simulink model "CryoDetHcd"  (R2016b)
settings: Solver=ode45  StartTime=0.0  StopTime=1e-3  RelTol=1e-3
PreLoadFcn:
  | setup_hcd
values from neighbouring files (symbols this model uses):
  A = sqrt(0.5*erfc(x))    [setup_hcd.m]
  Fadc = 307.2e6    (= 307200000)    [setupADCtoDACloopback.m]    (also in setupCryoFPGA_CMB.m; setup_hcd.m = 614000000)
undefined symbols (not defined in the file or in its folder): AXI4, B, C, D, etaRomData, freqRomData, freqRomData1, freqRomData2, freqRomData3, j, Lite
libraries: xbsIndex_r4 x897, CryoDetLibCMB x8, hdlsllib x8, dspsigops x2, simulink x1
(part 2 of 8)

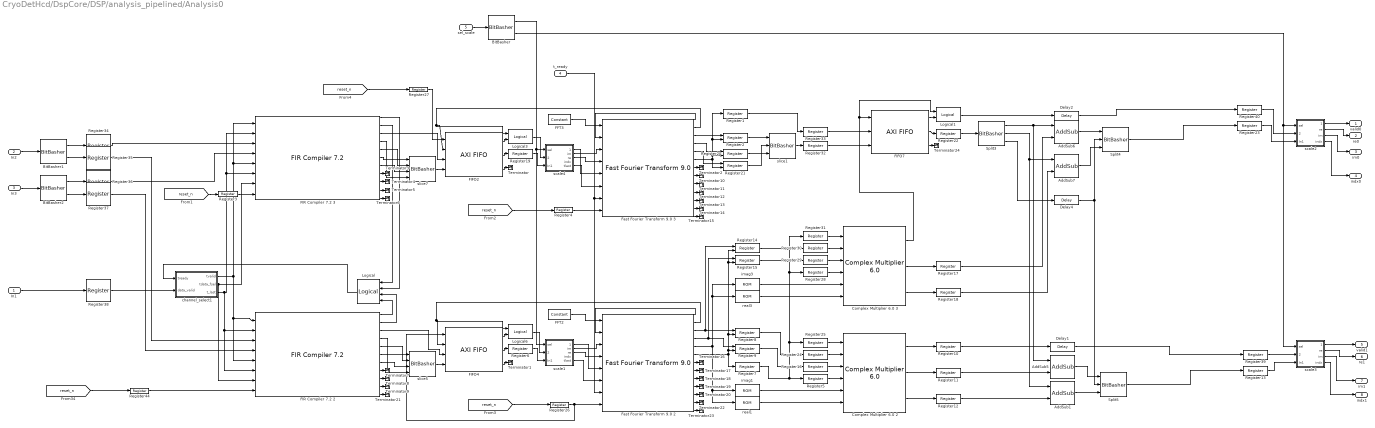
== system CryoDetHcd/DspCore/DSP/analysis_pipelined/Analysis0 ==
  In1 : Inport
  In2 : Inport  Port=2
  In3 : Inport  Port=3
  t_ready : Inport  Port=4
  sel_scale : Inport  Port=5
  AddSub{1,5..7} (4 alike) : xbsIndex_r4/AddSub  mode=Addition  use_carryin=off  use_carryout=off  en=off  latency=2  precision=Full  arith_type="Signed  (2's comp)"  n_bits=22  bin_pt=16  quantization=Truncate  overflow=Wrap  use_behavioral_HDL=on  hw_selection=Fabric  pipelined=off  dbl_ovrd=off  block_type=addsub
  BitBasher : xbsIndex_r4/BitBasher  bitexpr=|  display_expr=off  sr_1=sel0  arith_type1=Unsigned  bin_pt1=0  sr_2=sel1  arith_type2=Unsigned  bin_pt2=0  sr_3=3  arith_type3=Unsigned  bin_pt3=0  sr_4=4  arith_type4=Unsigned  bin_pt4=0  dbl_ovrd=off  block_type=bitbasher
      | sel0 = {in[0]}
      | sel1 = {in[1]}
  BitBasher1 : xbsIndex_r4/BitBasher  bitexpr=|  display_expr=off  sr_1=lo  arith_type1="Signed  (2's comp)"  bin_pt1=15  sr_2=hi  arith_type2="Signed  (2's comp)"  bin_pt2=15  sr_3=hi  arith_type3=Unsigned  bin_pt3=0  sr_4=4  arith_type4=Unsigned  bin_pt4=0  dbl_ovrd=off  block_type=bitbasher
      | lo = {in[15:0]}
      | hi = {in[31:16]}
  BitBasher2 : xbsIndex_r4/BitBasher  bitexpr=|  display_expr=off  sr_1=lo  arith_type1="Signed  (2's comp)"  bin_pt1=15  sr_2=hi  arith_type2="Signed  (2's comp)"  bin_pt2=15  sr_3=hi  arith_type3=Unsigned  bin_pt3=0  sr_4=4  arith_type4=Unsigned  bin_pt4=0  dbl_ovrd=off  block_type=bitbasher
      | lo = {in[15:0]}
      | hi = {in[31:16]}
  Complex Multiplier 6.0 2 : xbsIndex_r4/Complex Multiplier 6.0   hasatlast=off  hasatuser=off  atuserwidth=1  hasbtlast=off  hasbtuser=off  btuserwidth=1  multtype=Use_Mults  optimizegoal=Performance  flowcontrol=NonBlocking  outputwidth=24  roundmode=Truncate  hasctrltlast=off  hasctrltuser=off  ctrltuserwidth=1  outtlastbehv=Null  latencyconfig=Automatic  minimumlatency=34  aclken=off  aresetn=off  trim_axipin_name=on  simulation_type=hybrid_sim  simulation_model=sysgen:cmpy_v6_0  data_path_portlist={ 's_axis_a_tdata_real', 's_axis_a_tdata_imag', 's_axis_b_tdata_real', 's_axis_b_tdata_imag', 's_axis_ctrl_tdata_rounding_bit', 'm_axis_dout_tdata_real', 'm_axis_dout_tdata_imag' }  aportwidth=63  bportwidth=63  ip_name=Complex Multiplier  ip_version=6.0  dsptool_ready=true  ipcore_usecache=true  ipcore_useipmodelcache=true  ipcore_verbose=false  ipcore_latency_parameter='minimumlatency'  wrapper_available=true  port_translation_map={ 'aclken' => 'en', 'aresetn' => 'rst'}  block_type=cmpy_v6_0
  Complex Multiplier 6.0 3 : xbsIndex_r4/Complex Multiplier 6.0   hasatlast=off  hasatuser=off  atuserwidth=1  hasbtlast=off  hasbtuser=off  btuserwidth=1  multtype=Use_Mults  optimizegoal=Performance  flowcontrol=NonBlocking  outputwidth=24  roundmode=Truncate  hasctrltlast=off  hasctrltuser=off  ctrltuserwidth=1  outtlastbehv=Null  latencyconfig=Automatic  minimumlatency=34  aclken=off  aresetn=off  trim_axipin_name=on  simulation_type=hybrid_sim  simulation_model=sysgen:cmpy_v6_0  data_path_portlist={ 's_axis_a_tdata_real', 's_axis_a_tdata_imag', 's_axis_b_tdata_real', 's_axis_b_tdata_imag', 's_axis_ctrl_tdata_rounding_bit', 'm_axis_dout_tdata_real', 'm_axis_dout_tdata_imag' }  aportwidth=63  bportwidth=63  ip_name=Complex Multiplier  ip_version=6.0  dsptool_ready=true  ipcore_usecache=true  ipcore_useipmodelcache=true  ipcore_verbose=false  ipcore_latency_parameter='minimumlatency'  wrapper_available=true  port_translation_map={ 'aclken' => 'en', 'aresetn' => 'rst'}  block_type=cmpy_v6_0
  Delay1 : xbsIndex_r4/Delay  rst=off  infoeditControl=Selection of Reset will increase slice count due to use of real FFs and instead of SRLs  en=off  latency=2  reg_retiming=on  dbl_ovrd=off  block_type=delay
  Delay2 : xbsIndex_r4/Delay  rst=off  infoeditControl=Selection of Reset will increase slice count due to use of real FFs and instead of SRLs  en=off  latency=2  reg_retiming=on  dbl_ovrd=off  block_type=delay
  Delay4 : xbsIndex_r4/Delay  rst=off  infoeditControl=Selection of Reset will increase slice count due to use of real FFs and instead of SRLs  en=off  latency=2  reg_retiming=on  dbl_ovrd=off  block_type=delay
  FFT2 : xbsIndex_r4/Constant  const=1  gui_display_data_type=Fixed-point  arith_type=Unsigned  n_bits=1  bin_pt=0  preci_type=Single  exp_width=8  frac_width=24  explicit_period=off  period=1  equ=P=C  opselect=C  inp2=PCIN>>17  opr=+  inp1=P  carry=CIN  dbl_ovrd=off  block_type=constant
  FFT3 : xbsIndex_r4/Constant  const=1  gui_display_data_type=Fixed-point  arith_type=Unsigned  n_bits=1  bin_pt=0  preci_type=Single  exp_width=8  frac_width=24  explicit_period=off  period=1  equ=P=C  opselect=C  inp2=PCIN>>17  opr=+  inp1=P  carry=CIN  dbl_ovrd=off  block_type=constant
  FIFO2 : xbsIndex_r4/AXI FIFO  input_depth_axis=16  actual_fifo_depth_label=18  enable_tdata=on  enable_tdest=off  enable_tstrb=off  enable_tready=on  enable_tid=off  enable_tuser=off  enable_tkeep=off  enable_tlast=off  has_aresetn=on  enable_data_counts_axis=off  fifo_implementation_type_axis=Common Clock Distributed RAM  trim_axipin_name=on  programmable_full_type_axis=Full  full_threshold_assert_value_axis=0  programmable_empty_type_axis=Empty  empty_threshold_assert_value_axis=1022  underflow_flag_axi=0  underflow_sense_axi=Active High  overflow_flag_axi=0  overflow_sense_axi=Active High  block_type=axi_fifo
  FIFO4 : xbsIndex_r4/AXI FIFO  input_depth_axis=16  actual_fifo_depth_label=18  enable_tdata=on  enable_tdest=off  enable_tstrb=off  enable_tready=on  enable_tid=off  enable_tuser=off  enable_tkeep=off  enable_tlast=off  has_aresetn=on  enable_data_counts_axis=off  fifo_implementation_type_axis=Common Clock Distributed RAM  trim_axipin_name=on  programmable_full_type_axis=Full  full_threshold_assert_value_axis=0  programmable_empty_type_axis=Empty  empty_threshold_assert_value_axis=1022  underflow_flag_axi=0  underflow_sense_axi=Active High  overflow_flag_axi=0  overflow_sense_axi=Active High  block_type=axi_fifo
  FIFO7 : xbsIndex_r4/AXI FIFO  input_depth_axis=32  actual_fifo_depth_label=34  enable_tdata=on  enable_tdest=off  enable_tstrb=off  enable_tready=on  enable_tid=off  enable_tuser=off  enable_tkeep=off  enable_tlast=off  has_aresetn=off  enable_data_counts_axis=off  fifo_implementation_type_axis=Common Clock Distributed RAM  trim_axipin_name=on  programmable_full_type_axis=Full  full_threshold_assert_value_axis=0  programmable_empty_type_axis=Empty  empty_threshold_assert_value_axis=1022  underflow_flag_axi=0  underflow_sense_axi=Active High  overflow_flag_axi=0  overflow_sense_axi=Active High  block_type=axi_fifo
  FIR Compiler 7.2 2 : xbsIndex_r4/FIR Compiler 7.2   coefficientvector=analysis_coefficients2  coefficient_sets=8  coefficient_reload=off  filter_type=Single_Rate  rate_change_type=Integer  interpolation_rate=1  decimation_rate=1  zero_pack_factor=1  channel_sequence=Basic  number_channels=8  pattern_list='P4-0,P4-1,P4-2,P4-3,P4-4'  number_paths=2  ratespecification=Output_Sample_Period  sampleperiod=1.00000000  hardwareoversamplingrate=1  coefficient_sign=Signed  quantization=Quantize_Only  coefficient_width=25  bestprecision=on  coefficient_fractional_bits=28  coefficient_structure=Inferred  output_rounding_mode=Convergent_Rounding_to_Even  output_width=19  filter_architecture=Systolic_Multiply_Accumulate  optimization_goal=Area  optimization_list='None'  data_buffer_type=Automatic  coefficient_buffer_type=Automatic  input_buffer_type=Automatic  output_buffer_type=Automatic  preference_for_other_storage=Automatic  multi_column_support=Automatic  columnconfig='16'  inter_column_pipe_length=4  data_has_tlast=Vector_Framing  m_data_has_tready=off  s_data_has_fifo=off  s_data_has_tuser=Not_Required  m_data_has_tuser=Chan_ID_Field  s_config_sync_mode=On_Vector  s_config_method=By_Channel  num_reload_slots=1  has_aclken=off  has_aresetn=on  infoeditControl=ARESETn must be asserted for a minimum of 2 cycles  reset_data_vector=on  trim_axipin_name=on  simulation_type=hybrid_sim  simulation_model=sysgen:xfirv7_2_cmodel  data_path_portlist={ 's_axis_data_tdata', 'm_axis_data_tdata' }  passband_min=0.0  passband_max=0.5  stopband_min=0.5  stopband_max=1.0  filter_selection=1  gui_behaviour='Sysgen_GUI'  data_sign=Signed  data_width=16  data_fractional_bits=0  data_tuser_width=1  wrapper_available=true  ip_wrap_arbitrary_binary_point=true  ip_name=FIR Compiler  ip_version=7.2  dsptool_ready=true  ipcore_usecache=true  ipcore_useipmodelcache=true  port_translation_map={ 'aclken' => 'en', 'aresetn' => 'rst' }  run_core_at_system_period=true  ipcore_xco_need_fpga_part=true  block_type=fir_compiler_v7_2
      settings: infoedit=Maximum Possible : Maximizes oversampling rate. Abstracted input handshake (no s_data_tvalid) and automatic rate propagation.<br>Hardware Oversampling Rate : Specifies oversampling rate relative to the input sample period. Abstracted input handshake (no s_data_tvalid) and automatic rate propagation.<br>Input/Output Sample Period : Specifies absolute oversampling rate. No input handshake abstraction (exposes s_data_tvalid) and no rate propagation.
  FIR Compiler 7.2 3 : xbsIndex_r4/FIR Compiler 7.2   coefficientvector=analysis_coefficients1  coefficient_sets=8  coefficient_reload=off  filter_type=Single_Rate  rate_change_type=Integer  interpolation_rate=1  decimation_rate=1  zero_pack_factor=1  channel_sequence=Basic  number_channels=8  pattern_list='P4-0,P4-1,P4-2,P4-3,P4-4'  number_paths=2  ratespecification=Output_Sample_Period  sampleperiod=1.00000000  hardwareoversamplingrate=1  coefficient_sign=Signed  quantization=Quantize_Only  coefficient_width=25  bestprecision=on  coefficient_fractional_bits=28  coefficient_structure=Inferred  output_rounding_mode=Convergent_Rounding_to_Even  output_width=19  filter_architecture=Systolic_Multiply_Accumulate  optimization_goal=Area  optimization_list='None'  data_buffer_type=Automatic  coefficient_buffer_type=Automatic  input_buffer_type=Automatic  output_buffer_type=Automatic  preference_for_other_storage=Automatic  multi_column_support=Automatic  columnconfig='16'  inter_column_pipe_length=4  data_has_tlast=Vector_Framing  m_data_has_tready=off  s_data_has_fifo=off  s_data_has_tuser=Not_Required  m_data_has_tuser=Chan_ID_Field  s_config_sync_mode=On_Vector  s_config_method=By_Channel  num_reload_slots=1  has_aclken=off  has_aresetn=on  infoeditControl=ARESETn must be asserted for a minimum of 2 cycles  reset_data_vector=on  trim_axipin_name=on  simulation_type=hybrid_sim  simulation_model=sysgen:xfirv7_2_cmodel  data_path_portlist={ 's_axis_data_tdata', 'm_axis_data_tdata' }  passband_min=0.0  passband_max=0.5  stopband_min=0.5  stopband_max=1.0  filter_selection=1  gui_behaviour='Sysgen_GUI'  data_sign=Signed  data_width=16  data_fractional_bits=0  data_tuser_width=1  wrapper_available=true  ip_wrap_arbitrary_binary_point=true  ip_name=FIR Compiler  ip_version=7.2  dsptool_ready=true  ipcore_usecache=true  ipcore_useipmodelcache=true  port_translation_map={ 'aclken' => 'en', 'aresetn' => 'rst' }  run_core_at_system_period=true  ipcore_xco_need_fpga_part=true  block_type=fir_compiler_v7_2
      settings: infoedit=Maximum Possible : Maximizes oversampling rate. Abstracted input handshake (no s_data_tvalid) and automatic rate propagation.<br>Hardware Oversampling Rate : Specifies oversampling rate relative to the input sample period. Abstracted input handshake (no s_data_tvalid) and automatic rate propagation.<br>Input/Output Sample Period : Specifies absolute oversampling rate. No input handshake abstraction (exposes s_data_tvalid) and no rate propagation.
  Fast Fourier Transform 9.0 2 : xbsIndex_r4/Fast Fourier Transform 9.0   transform_length=8  target_clock_frequency=307  target_data_throughput=50  implementation_options=pipelined_streaming_io  run_time_configurable_transform_length=off  phase_factor_width=17  scaling_options=unscaled  rounding_modes=convergent_rounding  aclken=off  aresetn=on  output_ordering=natural_order  cyclic_prefix_insertion=off  throttle_scheme=nonrealtime  xk_index=on  ovflo=off  trim_axipin_name=on  memory_options_data=block_ram  memory_options_phase_factors=block_ram  number_of_stages_using_block_ram_for_data_and_phase_factors=0  memory_options_reorder=block_ram  memory_options_hybrid=off  complex_mult_type=use_mults_performance  butterfly_type=use_xtremedsp_slices  simulation_type=hybrid_sim  simulation_model=sysgen:xfftv9_cmodel  data_path_portlist={ 's_axis_data_tdata', 'm_axis_data_tdata', 'm_axis_status_tdata', 'event_fft_overflow' }  channels=1  input_ordering=natural_order  input_width=16  ip_name=Fast Fourier Transform  ip_version=9.0  dsptool_ready=true  ipcore_usecache=true  ipcore_useipmodelcache=true  wrapper_available=true  port_translation_map={ 'aclken' => 'en', 'aresetn' => 'rst'}  data_format=fixed_point  block_type=xfft_v9_0
  Fast Fourier Transform 9.0 3 : xbsIndex_r4/Fast Fourier Transform 9.0   transform_length=8  target_clock_frequency=307  target_data_throughput=50  implementation_options=pipelined_streaming_io  run_time_configurable_transform_length=off  phase_factor_width=17  scaling_options=unscaled  rounding_modes=convergent_rounding  aclken=off  aresetn=on  output_ordering=natural_order  cyclic_prefix_insertion=off  throttle_scheme=nonrealtime  xk_index=on  ovflo=off  trim_axipin_name=on  memory_options_data=block_ram  memory_options_phase_factors=block_ram  number_of_stages_using_block_ram_for_data_and_phase_factors=0  memory_options_reorder=block_ram  memory_options_hybrid=off  complex_mult_type=use_mults_performance  butterfly_type=use_xtremedsp_slices  simulation_type=hybrid_sim  simulation_model=sysgen:xfftv9_cmodel  data_path_portlist={ 's_axis_data_tdata', 'm_axis_data_tdata', 'm_axis_status_tdata', 'event_fft_overflow' }  channels=1  input_ordering=natural_order  input_width=16  ip_name=Fast Fourier Transform  ip_version=9.0  dsptool_ready=true  ipcore_usecache=true  ipcore_useipmodelcache=true  wrapper_available=true  port_translation_map={ 'aclken' => 'en', 'aresetn' => 'rst'}  data_format=fixed_point  block_type=xfft_v9_0
  Logical : xbsIndex_r4/Logical  logical_function=AND  inputs=4  en=off  latency=1  precision=Full  arith_type=Unsigned  n_bits=16  bin_pt=0  align_bp=on  dbl_ovrd=off  block_type=logical
  Logical1 : xbsIndex_r4/Logical  logical_function=AND  inputs=2  en=off  latency=1  precision=Full  arith_type=Unsigned  n_bits=16  bin_pt=0  align_bp=on  dbl_ovrd=off  block_type=logical
  Logical3 : xbsIndex_r4/Logical  logical_function=AND  inputs=2  en=off  latency=1  precision=Full  arith_type=Unsigned  n_bits=16  bin_pt=0  align_bp=on  dbl_ovrd=off  block_type=logical
  Logical6 : xbsIndex_r4/Logical  logical_function=AND  inputs=2  en=off  latency=1  precision=Full  arith_type=Unsigned  n_bits=16  bin_pt=0  align_bp=on  dbl_ovrd=off  block_type=logical
  Register{1,3..7,10..13,16..19,22..40,44} (34 alike) : xbsIndex_r4/Register  init=0  rst=off  en=off  dbl_ovrd=off  block_type=register
  Register{2,8..9,14..15,20..21} (7 alike) : xbsIndex_r4/Register  init=0  rst=off  en=on  dbl_ovrd=off  block_type=register
  Split3 : xbsIndex_r4/BitBasher  bitexpr=|  display_expr=off  sr_1=im  arith_type1="Signed  (2's comp)"  bin_pt1=17  sr_2=re  arith_type2="Signed  (2's comp)"  bin_pt2=17  sr_3=indx  arith_type3=Unsigned  bin_pt3=0  sr_4=4  arith_type4=Unsigned  bin_pt4=0  dbl_ovrd=off  block_type=bitbasher
      | im={in[43:22]}
      | re={in[21:0]}
      | indx = {in[46:44]}
  Split4 : xbsIndex_r4/BitBasher  bitexpr=out = {9'b0, indx, im, re}  display_expr=off  sr_1=out  arith_type1="Signed  (2's comp)"  bin_pt1=0  sr_2=im  arith_type2="Signed  (2's comp)"  bin_pt2=18  sr_3=3  arith_type3=Unsigned  bin_pt3=0  sr_4=4  arith_type4=Unsigned  bin_pt4=0  dbl_ovrd=off  block_type=bitbasher
  Split5 : xbsIndex_r4/BitBasher  bitexpr=out = {9'b0, indx, im, re}  display_expr=off  sr_1=out  arith_type1="Signed  (2's comp)"  bin_pt1=0  sr_2=im  arith_type2="Signed  (2's comp)"  bin_pt2=18  sr_3=3  arith_type3=Unsigned  bin_pt3=0  sr_4=4  arith_type4=Unsigned  bin_pt4=0  dbl_ovrd=off  block_type=bitbasher
  Terminator{,1..24} (25 alike) : Terminator
  channel_select1 : Subsystem
  imag1 : xbsIndex_r4/ROM  depth=8  initVector=imag(exp(-j*2*pi*(8:15)/16))  distributed_mem=Block RAM  rst=off  init_reg=0  en=off  latency=2  gui_display_data_type=Fixed-point  arith_type="Signed  (2's comp)"  n_bits=18  bin_pt=16  preci_type=Single  exp_width=8  frac_width=24  optimize=Area  use_rpm=on  dbl_ovrd=off  block_type=sprom
  imag3 : xbsIndex_r4/ROM  depth=8  initVector=imag(exp(-j*2*pi*(0:7)/16))  distributed_mem=Block RAM  rst=off  init_reg=0  en=off  latency=2  gui_display_data_type=Fixed-point  arith_type="Signed  (2's comp)"  n_bits=18  bin_pt=16  preci_type=Single  exp_width=8  frac_width=24  optimize=Area  use_rpm=on  dbl_ovrd=off  block_type=sprom
  real1 : xbsIndex_r4/ROM  depth=8  initVector=real(exp(-j*2*pi*(8:15)/16))  distributed_mem=Block RAM  rst=off  init_reg=0  en=off  latency=2  gui_display_data_type=Fixed-point  arith_type="Signed  (2's comp)"  n_bits=18  bin_pt=16  preci_type=Single  exp_width=8  frac_width=24  optimize=Area  use_rpm=on  dbl_ovrd=off  block_type=sprom
  real3 : xbsIndex_r4/ROM  depth=8  initVector=real(exp(-j*2*pi*(0:7)/16))  distributed_mem=Block RAM  rst=off  init_reg=0  en=off  latency=2  gui_display_data_type=Fixed-point  arith_type="Signed  (2's comp)"  n_bits=18  bin_pt=16  preci_type=Single  exp_width=8  frac_width=24  optimize=Area  use_rpm=on  dbl_ovrd=off  block_type=sprom
  scale1 : Subsystem
  scale2 : Subsystem
  scale3 : Subsystem
  scale4 : Subsystem
  slice1 : xbsIndex_r4/BitBasher  bitexpr="out ={17'b0,  indx, im, re }"  display_expr=off  sr_1=out  arith_type1=Unsigned  bin_pt1=0  sr_2=2  arith_type2="Signed  (2's comp)"  bin_pt2=16  sr_3=3  arith_type3=Unsigned  bin_pt3=0  sr_4=4  arith_type4=Unsigned  bin_pt4=0  dbl_ovrd=off  block_type=bitbasher
  slice5 : xbsIndex_r4/BitBasher  bitexpr=out ={19'b0, tlast, indx, im[20:0], re[20:0] }  display_expr=off  sr_1=out  arith_type1=Unsigned  bin_pt1=0  sr_2=2  arith_type2="Signed  (2's comp)"  bin_pt2=16  sr_3=3  arith_type3=Unsigned  bin_pt3=0  sr_4=4  arith_type4=Unsigned  bin_pt4=0  dbl_ovrd=off  block_type=bitbasher
  slice7 : xbsIndex_r4/BitBasher  bitexpr=out ={19'b0, tlast, indx, im[20:0], re[20:0] }  display_expr=off  sr_1=out  arith_type1=Unsigned  bin_pt1=0  sr_2=2  arith_type2="Signed  (2's comp)"  bin_pt2=16  sr_3=3  arith_type3=Unsigned  bin_pt3=0  sr_4=4  arith_type4=Unsigned  bin_pt4=0  dbl_ovrd=off  block_type=bitbasher
  valid0 : Outport
  re0 : Outport  Port=2
  im0 : Outport  Port=3
  indx0 : Outport  Port=4
  valid1 : Outport  Port=5
  re1 : Outport  Port=6
  im1 : Outport  Port=7
  indx1 : Outport  Port=8
  wires:
  Register33/1 -> FIFO7/2
  Register32/1 -> FIFO7/3
  channel_select1/2(tdata_fsel) -> FIR Compiler 7.2 2/7, FIR Compiler 7.2 3/7
  channel_select1/1(tvalid) -> FIR Compiler 7.2 3/5, FIR Compiler 7.2 3/1, FIR Compiler 7.2 2/5, FIR Compiler 7.2 2/1
  In3/1 -> BitBasher2/1
  In1/1 -> Register38/1
  Logical/1 -> channel_select1/1(tready)
  FIR Compiler 7.2 2/7 -> slice5/3
  FIR Compiler 7.2 2/5 -> slice5/2
  FIFO4/1 -> Logical6/2
  Fast Fourier Transform 9.0 2/2 -> FIFO4/2, Logical6/1
  FIFO4/2 -> Register6/1
  Register6/1 -> scale1/3(In1)
  Logical6/1 -> scale1/2(valid_i)
  FIR Compiler 7.2 2/4 -> slice5/4
  FFT2/1 -> Fast Fourier Transform 9.0 2/1
  Fast Fourier Transform 9.0 2/1 -> Fast Fourier Transform 9.0 2/2
  Fast Fourier Transform 9.0 2/3 -> Register14/1, Register8/1
  Fast Fourier Transform 9.0 2/4 -> Register15/1, Register9/1
  Fast Fourier Transform 9.0 2/6 -> Register8/2, Register14/2, Register15/2, Register9/2, Register7/1
  Register9/1 -> Register16/1
  Register8/1 -> Register24/1
  Register7/1 -> Register28/1, Register31/1, Register25/1, Register5/1
  Complex Multiplier 6.0 2/3 -> Register12/1
  Complex Multiplier 6.0 2/2 -> Register11/1
  Complex Multiplier 6.0 2/1 -> Register10/1
  Register12/1 -> AddSub1/2
  Register11/1 -> AddSub5/2
  Register10/1 -> Delay1/1
  AddSub5/1 -> Split5/1
  AddSub1/1 -> Split5/3
  Split5/1 -> Register13/1
  Register15/1 -> Register29/1
  Register14/1 -> Register30/1
  Complex Multiplier 6.0 3/1 -> Logical1/1, FIFO7/1
  Complex Multiplier 6.0 3/2 -> Register17/1
  Complex Multiplier 6.0 3/3 -> Register18/1
  FIR Compiler 7.2 2/1 -> Logical/4
  FIR Compiler 7.2 2/2 -> Logical/3
  FIR Compiler 7.2 3/1 -> Logical/2
  FIR Compiler 7.2 3/2 -> Logical/1
  FIR Compiler 7.2 3/6 -> slice7/1
  FIR Compiler 7.2 3/7 -> slice7/3
  FIR Compiler 7.2 3/5 -> slice7/2
  FIR Compiler 7.2 3/4 -> slice7/4
  FIR Compiler 7.2 3/8 -> Terminator3/1
  FIR Compiler 7.2 3/9 -> Terminator4/1
  FIR Compiler 7.2 3/10 -> Terminator5/1
  FIR Compiler 7.2 3/11 -> Terminator6/1
  FIR Compiler 7.2 2/8 -> Terminator7/1
  FIR Compiler 7.2 2/9 -> Terminator8/1
  FIR Compiler 7.2 2/10 -> Terminator9/1
  FIR Compiler 7.2 2/11 -> Terminator21/1
  Fast Fourier Transform 9.0 3/2 -> FIFO2/2, Logical3/1
  FIFO2/2 -> Register19/1
  Register19/1 -> scale4/3(In1)
  FFT3/1 -> Fast Fourier Transform 9.0 3/1
  Fast Fourier Transform 9.0 3/1 -> Fast Fourier Transform 9.0 3/2
  scale4/5(tlast) -> Fast Fourier Transform 9.0 3/6
  channel_select1/3(t_last) -> FIR Compiler 7.2 3/2, FIR Compiler 7.2 3/6, FIR Compiler 7.2 2/6, FIR Compiler 7.2 2/2
  Fast Fourier Transform 9.0 3/3 -> Register2/1
  Fast Fourier Transform 9.0 3/4 -> Register20/1
  Fast Fourier Transform 9.0 3/6 -> Register1/1, Register2/2, Register20/2, Register21/2
  Fast Fourier Transform 9.0 3/5 -> Register21/1
  Register2/1 -> slice1/1
  Register21/1 -> slice1/2
  Register20/1 -> slice1/3
  Register1/1 -> Register33/1
  slice1/1 -> Register32/1
  FIFO7/2 -> Register22/1
  FIFO7/1 -> Logical1/2
  Register22/1 -> Split3/1
  Split3/1 -> AddSub5/1, AddSub6/1
  Split3/2 -> AddSub1/1, AddSub7/1
  Register17/1 -> AddSub6/2
  Register18/1 -> AddSub7/2
  Logical1/1 -> Delay2/1
  Delay4/1 -> Split5/2, Split4/2
  AddSub6/1 -> Split4/1
  AddSub7/1 -> Split4/3
  Delay2/1 -> Register40/1
  Register40/1 -> scale2/2(valid_i)
  scale2/2(re) -> re0/1
  scale2/4(indx) -> indx0/1
  Split4/1 -> Register23/1
  Split3/3 -> Delay4/1
  FIFO2/3 -> Terminator/1
  FIFO4/3 -> Terminator1/1
  Fast Fourier Transform 9.0 3/7 -> Terminator2/1
  Fast Fourier Transform 9.0 3/8 -> Terminator10/1
  Fast Fourier Transform 9.0 3/9 -> Terminator11/1
  Fast Fourier Transform 9.0 3/10 -> Terminator12/1
  Fast Fourier Transform 9.0 3/11 -> Terminator13/1
  Fast Fourier Transform 9.0 3/12 -> Terminator14/1
  Fast Fourier Transform 9.0 3/13 -> Terminator15/1
  Fast Fourier Transform 9.0 2/7 -> Terminator16/1
  Fast Fourier Transform 9.0 2/8 -> Terminator17/1
  Fast Fourier Transform 9.0 2/9 -> Terminator18/1
  Fast Fourier Transform 9.0 2/10 -> Terminator19/1
  Fast Fourier Transform 9.0 2/11 -> Terminator20/1
  Fast Fourier Transform 9.0 2/12 -> Terminator22/1
  Fast Fourier Transform 9.0 2/13 -> Terminator23/1
  FIFO7/3 -> Terminator24/1
  FIFO2/1 -> Logical3/2
  Fast Fourier Transform 9.0 2/5 -> real1/1, imag1/1, real3/1, imag3/1
  FIR Compiler 7.2 2/6 -> slice5/1
  real1/1 -> Complex Multiplier 6.0 2/6
  imag1/1 -> Complex Multiplier 6.0 2/5
  Register5/1 -> Complex Multiplier 6.0 2/4
  Register16/1 -> Complex Multiplier 6.0 2/3
  Register24/1 -> Complex Multiplier 6.0 2/2
  Register25/1 -> Complex Multiplier 6.0 2/1
  real3/1 -> Complex Multiplier 6.0 3/6
  imag3/1 -> Complex Multiplier 6.0 3/5
  Register28/1 -> Complex Multiplier 6.0 3/4
  Register29/1 -> Complex Multiplier 6.0 3/3
  Register30/1 -> Complex Multiplier 6.0 3/2
  Register31/1 -> Complex Multiplier 6.0 3/1
  In2/1 -> BitBasher1/1
  Register34/1 -> FIR Compiler 7.2 3/3
  Register35/1 -> FIR Compiler 7.2 2/3
  Register36/1 -> FIR Compiler 7.2 3/4
  Register37/1 -> FIR Compiler 7.2 2/4
  Register38/1 -> channel_select1/2(data_valid)
  BitBasher1/1 -> Register34/1
  BitBasher1/2 -> Register35/1
  BitBasher2/1 -> Register36/1
  BitBasher2/2 -> Register37/1
  scale4/3(re) -> Fast Fourier Transform 9.0 3/4
  scale4/2(im) -> Fast Fourier Transform 9.0 3/3
  scale4/1(valid_o) -> Fast Fourier Transform 9.0 3/5
  Logical3/1 -> scale4/2(valid_i)
  scale1/5(tlast) -> Fast Fourier Transform 9.0 2/6
  scale1/1(valid_o) -> Fast Fourier Transform 9.0 2/5
  scale1/2(im) -> Fast Fourier Transform 9.0 2/3
  scale1/3(re) -> Fast Fourier Transform 9.0 2/4
  BitBasher/2 -> scale2/1(sel), scale3/1(sel)
  scale2/3(im) -> im0/1
  Register23/1 -> scale2/3(In1)
  scale2/1(valid_o) -> valid0/1
  Register39/1 -> scale3/2(valid_i)
  Register13/1 -> scale3/3(In1)
  scale3/1(valid_o) -> valid1/1
  scale3/2(re) -> re1/1
  scale3/3(im) -> im1/1
  scale3/4(indx) -> indx1/1
  sel_scale/1 -> BitBasher/1
  BitBasher/1 -> scale1/1(sel), scale4/1(sel)
  [reset_n] -> Register44/1
  [reset_n] -> Register3/1
  [reset_n] -> Register4/1
  [reset_n] -> Register26/1
  Register44/1 -> FIR Compiler 7.2 2/8
  Register3/1 -> FIR Compiler 7.2 3/8
  Register4/1 -> Fast Fourier Transform 9.0 3/8
  Register26/1 -> FIFO4/1, Fast Fourier Transform 9.0 2/8
  slice7/1 -> FIFO2/4
  FIR Compiler 7.2 3/3 -> FIFO2/3
  [reset_n] -> Register27/1
  Register27/1 -> FIFO2/1
  slice5/1 -> FIFO4/4
  FIR Compiler 7.2 2/3 -> FIFO4/3
  Delay1/1 -> Register39/1
  t_ready/1 -> Fast Fourier Transform 9.0 2/7, Fast Fourier Transform 9.0 3/7
